simulink model "Drone_2M_sim"  (R2021b)
settings: Solver=VariableStepAuto  StartTime=0.0  StopTime=5  RelTol=1e-3
values from neighbouring files (symbols this model uses):
  N = N + 1    (= 1)    [findp.m]    (also in findpd.m = N0; findpi.m; findpid.m)
undefined symbols (not defined in the file or in its folder): batteryMass, batVolt, body, deadCurrent, Dist, footZ, h1al, h1iuse, h1kp, h1td, h1ti, hoverControl, hoverVoltage, hval, hviuse, hvkp, hvtd, hvti, KDrag, Km, Ktrust, minimumMotorVolt, motorMass, paal, pakp, patd, pati, pitch_act_lim, propellerMass, pv_iuse, pval, pvkp, pvtd, pvti, Ra, raal, rakp, ral, ratd, rati, rkp, roll_act_lim, roll_limit, rtd, servoUs2Rad, trust_lim, TubeMasse, TubeX, TubeY, UKp, ULimit, UTau_h, X, xal, xkp, xtd, xti, xtiUse, xval, xvkp ... (+27)
libraries: sm_lib x86, nesl_utility x39, sharedtransform x1
(part 4 of 4)

== system Drone_2M_sim/Control units/height_control/height vel ctrl ==
  ref : Inport
  measurement : Inport  Port=2
  Constant : Constant  Value=hoverControl
  Gain : Gain  Gain=hvkp
  Gain1 : Gain  Gain=hviuse/hvti
  Integrator : Integrator  InitialConditionSource=external  InitialCondition=minimumMotorVolt  LimitOutput=on  UpperSaturationLimit=1000  LowerSaturationLimit=-1000
  Mux1 : Mux  Inputs=3
  Mux3 : Mux
  Saturation6 : Saturate  UpperLimit=trust_lim  LowerLimit=0
  Sum : Sum  Inputs=|+-
  Sum1 : Sum  Inputs=|++
  Transfer Fcn : TransferFcn  Numerator=[hvtd 1]  Denominator=[hval*hvtd 1]
  height-control-in : Scope
  height-control-out : Scope
  u : Outport  VectorParamsAs1DForOutWhenUnconnected=off
  wires:
  ref/1 -> Mux3/4, Sum/1  "ref"
  measurement/1 -> Mux3/2, Transfer Fcn/1  "m1"
  Sum/1 -> Mux3/1, Gain/1  "e"
  Integrator/1 -> Sum1/1, Mux1/1  "i"
  Gain1/1 -> Integrator/1
  Mux3/1 -> height-control-in/1
  Saturation6/1 -> Mux1/3, u/1  "u"
  Gain/1 -> Sum1/2, Mux1/2, Gain1/1  "eKp"
  Mux1/1 -> height-control-out/1
  Sum1/1 -> Saturation6/1
  Transfer Fcn/1 -> Mux3/3, Sum/2  "m2"
  Constant/1 -> Integrator/2

== system Drone_2M_sim/Control units/yaw ctrl/angle_lin_pm_pi ==
  rad-in : Inport
  Atan2 : Trigonometry  Operator=atan2
  Sin : Trigonometry
  Sin1 : Trigonometry  Operator=cos
  rad-out : Outport
  wires:
  Atan2/1 -> rad-out/1
  Sin/1 -> Atan2/1
  rad-in/1 -> Sin/1, Sin1/1
  Sin1/1 -> Atan2/2
